simulink model "testAlphaCeiling"  (R2018b)
settings: Solver=VariableStepDiscrete  StartTime=0.0  StopTime=10  RelTol=1e-3  EnableMultiTasking=on
libraries: carnot x2, simulink x1
settings Model: Creator=drhf  LastModifiedBy=drhf
settings DataIOCC: LimitDataPoints=on  SaveFormat=Array  ReturnWorkspaceOutputs=on
settings OptimizationCC: DefaultParameterBehavior=Inlined  LifeSpan=inf
settings DebuggingCC: ReadBeforeWriteMsg=DisableAll  WriteAfterWriteMsg=DisableAll  WriteAfterReadMsg=DisableAll  UnderspecifiedInitializationDetection=Classic  MergeDetectMultiDrivingBlocksExec=none  SolverPrmCheckMsg=warning  MultiTaskDSMMsg=none  SFUnexpectedBacktrackingDiag=warning  SFNoUnconditionalDefaultTransitionDiag=warning  SFExecutionAtInitializationDiag=none
settings HardwareCC: ProdBitPerPointer=32  ProdBitPerSizeT=32  ProdBitPerPtrDiffT=32  ProdLargestAtomicFloat=None  ProdIntDivRoundTo=Undefined  ProdEndianess=Unspecified  ProdWordSize=32  ProdHWDeviceType=32-bit Generic
settings ModelReferenceCC: UpdateModelReferenceTargets=IfOutOfDate  PropagateSignalLabelsOutOfModel=off
settings SFSimCC: SFSimEcho=off  SimUseLocalCustomCode=off
settings RTWCC: RTWUseLocalCustomCode=off
settings CodeAppCC: StateflowObjectComments=on
settings GRTTargetCC: TargetLangStandard=C89/C90 (ANSI)  GeneratePreprocessorConditionals=Disable all
settings ConfigComp: CovMetricSettings=dw  CovHtmlReporting=on  CovSaveCumulativeToWorkspaceVar=on  CovSaveSingleToWorkspaceVar=on  CovExternalEMLEnable=off

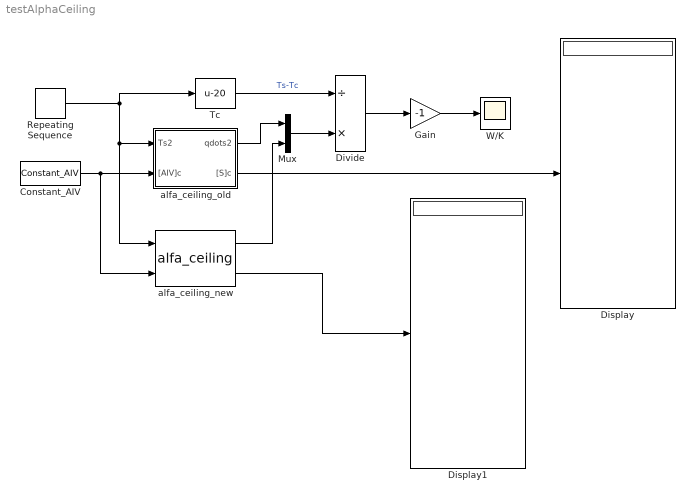
== system testAlphaCeiling ==
  Constant_AIV : carnot/Source/Ventilation/Constant_AIV  Tsens=20  Tcon=20  Trad=20  mw=0.012  mco=0.01  rhoair=1.2  cpair=1004  pair=100000  nair=0.5
  Display : Display
  Display1 : Display
  Divide : Product  Inputs=/*
  Gain : Gain  Gain=-1
  Mux : Mux  Inputs=2
  Repeating Sequence : simulink/Sources/Repeating Sequence  rep_seq_t=[0 10]  rep_seq_y=[10 30]
  Tc : Bias  Bias=-20
  W/K : Scope
  alfa_ceiling_new : carnot/Basic/Heat_Transfer/alfa_ceiling  active=0  emission_c=0.65  wallsurface=1
  alfa_ceiling_old : Subsystem  mask(ALFA){active=0, emission_c=0.65, wallsurface=1}
      mask prompts: active "active layer (0 / 1)"; emission_c "lonwave emissivity of surface (0..1)"; wallsurface "Ceiling surface in m²"
      mask help:
      | Convective and radiative heat transfer at the SURFACE OF A HORIZONTAL CEELING.
      | [AIV] : conditions of zone node,
      | Ts : temperature of outdoor wall surface, °C,
      | qdots : specific heat flow into wall construction, W/m^2,
      | [S] : heat and air flow to zone node.
  wires:
  Constant_AIV/1 -> alfa_ceiling_old/2("[AIV]c"), alfa_ceiling_new/2
  Repeating Sequence/1 -> alfa_ceiling_old/1(Ts2), alfa_ceiling_new/1, Tc/1
  alfa_ceiling_old/2("[S]c") -> Display/1
  alfa_ceiling_new/2 -> Display1/1
  Tc/1 -> Divide/1  "Ts-Tc"
  alfa_ceiling_new/1 -> Mux/2
  alfa_ceiling_old/1(qdots2) -> Mux/1
  Mux/1 -> Divide/2
  Divide/1 -> Gain/1
  Gain/1 -> W/K/1

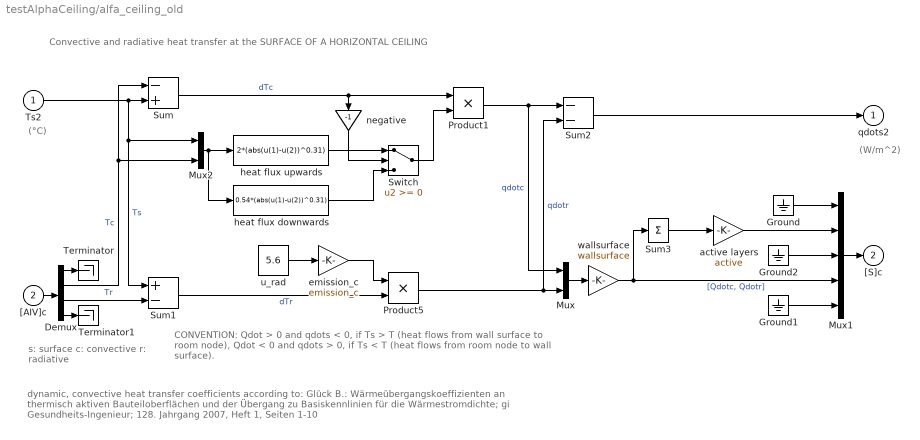
== system testAlphaCeiling/alfa_ceiling_old ==
  note: (°C)
  note: (W/m^2)
  note: Convective and radiative heat transfer at the SURFACE OF A HORIZONTAL CEILING
  note: s: surface
      | c: convective
      | r: radiative
  note: CONVENTION:
      | Qdot > 0 and qdots < 0, if Ts > T (heat flows from wall surface to room node),
      | Qdot < 0 and qdots > 0, if Ts < T (heat flows from room node to wall surface).
  note: dynamic, convective heat transfer coefficients according to: Glück B.: Wärmeübergangskoeffizienten an thermisch aktiven Bauteiloberflächen
      | und der Übergang zu Basiskennlinien für die Wärmestromdichte; gi Gesundheits-Ingenieur; 128. Jahrgang 2007, Heft 1, Seiten 1-10
  Ts2 : Inport
  "[AIV]c" : Inport  Port=2
  Demux : Demux  Outputs=[1 1 1 6]
  Ground : Ground
  Ground1 : Ground
  Ground2 : Ground
  Mux : Mux  Inputs=[1 1]
  Mux1 : Mux  Inputs=[4 1 1 2 5]
  Mux2 : Mux  Inputs=2
  Product1 : Product  SaturateOnIntegerOverflow=on  RndMeth=Zero  InputSameDT=on  OutDataTypeStr=Inherit: Same as first input
  Product5 : Product  SaturateOnIntegerOverflow=on  RndMeth=Zero  InputSameDT=on  OutDataTypeStr=Inherit: Same as first input
  Sum : Sum  Inputs=-+  SaturateOnIntegerOverflow=on  InputSameDT=on  OutDataTypeStr=Inherit: Same as first input
  Sum1 : Sum  Inputs=+-  SaturateOnIntegerOverflow=on  InputSameDT=on  OutDataTypeStr=Inherit: Same as first input
  Sum2 : Sum  Inputs=--  SaturateOnIntegerOverflow=on  InputSameDT=on  OutDataTypeStr=Inherit: Same as first input
  Sum3 : Sum  Inputs=1  SaturateOnIntegerOverflow=on  InputSameDT=on  OutDataTypeStr=Inherit: Same as first input
  Switch : Switch
  Terminator : Terminator
  Terminator1 : Terminator
  active layers : Gain  Gain=active  SaturateOnIntegerOverflow=on  OutDataTypeStr=Inherit: Same as input  ParamDataTypeStr=Inherit: Same as input
  emission_c : Gain  Gain=emission_c  SaturateOnIntegerOverflow=on  OutDataTypeStr=Inherit: Same as input  ParamDataTypeStr=Inherit: Same as input
  heat flux downwards : Fcn  Expr=0.54*(abs(u(1)-u(2))^0.31)
  heat flux upwards : Fcn  Expr=2*(abs(u(1)-u(2))^0.31)
  negative : Gain  Gain=-1  SaturateOnIntegerOverflow=on  OutDataTypeStr=Inherit: Same as input  ParamDataTypeStr=Inherit: Same as input
  u_rad : Constant  Value=5.6
  wallsurface : Gain  Gain=wallsurface  SaturateOnIntegerOverflow=on  OutDataTypeStr=Inherit: Same as input  ParamDataTypeStr=Inherit: Same as input
  qdots2 : Outport
  "[S]c" : Outport  Port=2
  wires:
  active layers/1 -> Mux1/2
  Ground2/1 -> Mux1/3
  Mux1/1 -> "[S]c"/1
  Ground1/1 -> Mux1/5
  Ground/1 -> Mux1/1
  Sum3/1 -> active layers/1
  wallsurface/1 -> Sum3/1, Mux1/4  "[Qdotc, Qdotr]"
  Ts2/1 -> Sum/2, Sum1/1, Mux2/1  "Ts"
  u_rad/1 -> emission_c/1
  Demux/2 -> Sum/1, Mux2/2  "Tc"
  Mux/1 -> wallsurface/1
  Product5/1 -> Mux/2, Sum2/2  "qdotr"
  emission_c/1 -> Product5/1
  Sum1/1 -> Product5/2  "dTr"
  Demux/1 -> Terminator/1
  "[AIV]c"/1 -> Demux/1
  Demux/4 -> Terminator1/1
  Sum2/1 -> qdots2/1
  Product1/1 -> Mux/1, Sum2/1  "qdotc"
  Sum/1 -> Product1/1, negative/1  "dTc"
  Demux/3 -> Sum1/2  "Tr"
  Mux2/1 -> heat flux upwards/1, heat flux downwards/1
  Switch/1 -> Product1/2
  heat flux upwards/1 -> Switch/1
  heat flux downwards/1 -> Switch/3
  negative/1 -> Switch/2
